simulink model "Testing"  (R2018b)
settings: Solver=VariableStepAuto  StartTime=0.0  StopTime=10.0  RelTol=1e-3
undefined symbols (not defined in the file): BattTempBp, BM_TiCtctrCnct_P, BM_TiCtctrDCnct_P, BMS_EnaFltSts, BMS_ModeEnaFltChk, BMS_TiSample_C, BPC_BattTotalCharge_P, BPC_BattTotalEnergy_P, CapLUTBp, CapSOCBp, CVM_DMaxVCellMaxCutoff_P, CVM_DMaxVCellMaxDrtd_P, CVM_DMaxVCellMaxWarn_P, CVM_DMaxVCellMinCutoff_P, CVM_DMaxVCellMinDrtd_P, CVM_DMaxVCellMinWarn_P, CVM_DMinVCellMaxCutoff_P, CVM_DMinVCellMaxDrtd_P, CVM_DMinVCellMaxWarn_P, CVM_DMinVCellMinCutoff_P, CVM_DMinVCellMinDrtd_P, CVM_DMinVCellMinWarn_P, CVM_VCellMaxCutoffTh_P, CVM_VCellMaxDrtdTh_P, CVM_VCellMaxWarnTh_P, CVM_VCellMinCutoffTh_P, CVM_VCellMinDrtdTh_P, CVM_VCellMinWarnTh_P, DiscIntNeverNeededParam, Em, MTM_DMaxTMdulMaxCutoff_P, MTM_DMaxTMdulMaxDrtd_P, MTM_DMaxTMdulMaxWarn_P, MTM_DMaxTMdulMinCutoff_P, MTM_DMaxTMdulMinDrtd_P, MTM_DMaxTMdulMinWarn_P, MTM_DMinTMdulMaxCutoff_P, MTM_DMinTMdulMaxDrtd_P, MTM_DMinTMdulMaxWarn_P, MTM_DMinTMdulMinCutoff_P, MTM_DMinTMdulMinDrtd_P, MTM_DMinTMdulMinWarn_P, MTM_TMdulMaxCutoffTh_P, MTM_TMdulMaxDrtdTh_P, MTM_TMdulMaxWarnTh_P, MTM_TMdulMinCutoffTh_P, MTM_TMdulMinDrtdTh_P, MTM_TMdulMinWarnTh_P, NrCutoff_C, NrDrtd_C, NrNoFlt_C, NrTMdulSnsr_C, NrWarn_C, RInt
libraries: BMSLib x12
settings Model: Creator=Administrator  LastModifiedBy=Administrator
settings OptimizationCC: DefaultUnderspecifiedDataType=single

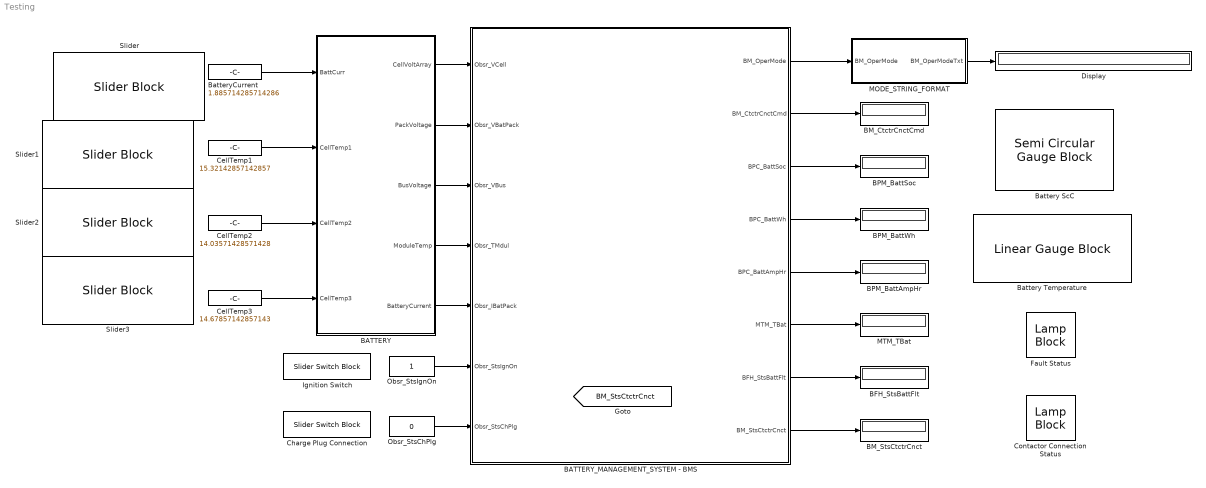
== system Testing ==
  BATTERY : Subsystem
  BATTERY_MANAGEMENT_SYSTEM - BMS : Subsystem
  BFH_StsBattFlt : Display
  BM_CtctrCnctCmd : Display
  BM_StsCtctrCnct : Display
  BPM_BattAmpHr : Display
  BPM_BattSoc : Display
  BPM_BattWh : Display
  Battery ScC : SemiCircularGaugeBlock  WebBlockId=770
  Battery Temperature : LinearGaugeBlock  WebBlockId=771  ScaleMin=-60  ScaleMax=60
  BatteryCurrent : Constant  Value=1.885714285714286  OutDataTypeStr=double
  CellTemp1 : Constant  Value=15.32142857142857  OutDataTypeStr=double
  CellTemp2 : Constant  Value=14.03571428571428  OutDataTypeStr=double
  CellTemp3 : Constant  Value=14.67857142857143  OutDataTypeStr=double
  Charge Plug Connection : SliderSwitchBlock  WebBlockId=776
      settings: Values={{'Off', 'On'}, [0 1]}
  Contactor Connection Status : LampBlock  WebBlockId=777
  Display : Display
  Fault Status : LampBlock  WebBlockId=779
  Ignition Switch : SliderSwitchBlock  WebBlockId=781
      settings: Values={{'Off', 'On'}, [0 1]}
  MODE_STRING_FORMAT : Subsystem
  MTM_TBat : Display
  Obsr_StsChPlg : Constant  Value=0  OutDataTypeStr=boolean
  Obsr_StsIgnOn : Constant  OutDataTypeStr=boolean
  Slider : SliderBlock  WebBlockId=791  ScaleMin=-24  ScaleMax=24
  Slider1 : SliderBlock  WebBlockId=792  ScaleMin=-30  ScaleMax=60
  Slider2 : SliderBlock  WebBlockId=793  ScaleMin=-30  ScaleMax=60
  Slider3 : SliderBlock  WebBlockId=794  ScaleMin=-30  ScaleMax=60
  tag scope: BM_StsCtctrCnct=global
  wires:
  Obsr_StsChPlg/1 -> BATTERY_MANAGEMENT_SYSTEM - BMS/7(Obsr_StsChPlg)
  BATTERY_MANAGEMENT_SYSTEM - BMS/2(BM_CtctrCnctCmd) -> BM_CtctrCnctCmd/1
  BATTERY_MANAGEMENT_SYSTEM - BMS/3(BPC_BattSoc) -> BPM_BattSoc/1
  BatteryCurrent/1 -> BATTERY/1(BattCurr)
  Obsr_StsIgnOn/1 -> BATTERY_MANAGEMENT_SYSTEM - BMS/6(Obsr_StsIgnOn)
  MODE_STRING_FORMAT/1(BM_OperModeTxt) -> Display/1
  BATTERY/2(PackVoltage) -> BATTERY_MANAGEMENT_SYSTEM - BMS/2(Obsr_VBatPack)
  BATTERY_MANAGEMENT_SYSTEM - BMS/1(BM_OperMode) -> MODE_STRING_FORMAT/1(BM_OperMode)
  BATTERY_MANAGEMENT_SYSTEM - BMS/4(BPC_BattWh) -> BPM_BattWh/1
  BATTERY_MANAGEMENT_SYSTEM - BMS/5(BPC_BattAmpHr) -> BPM_BattAmpHr/1
  CellTemp1/1 -> BATTERY/2(CellTemp1)
  BATTERY/5(BatteryCurrent) -> BATTERY_MANAGEMENT_SYSTEM - BMS/5(Obsr_IBatPack)
  BATTERY/4(ModuleTemp) -> BATTERY_MANAGEMENT_SYSTEM - BMS/4(Obsr_TMdul)
  CellTemp3/1 -> BATTERY/4(CellTemp3)
  CellTemp2/1 -> BATTERY/3(CellTemp2)
  BATTERY/1(CellVoltArray) -> BATTERY_MANAGEMENT_SYSTEM - BMS/1(Obsr_VCell)
  BATTERY_MANAGEMENT_SYSTEM - BMS/6(MTM_TBat) -> MTM_TBat/1
  BATTERY_MANAGEMENT_SYSTEM - BMS/7(BFH_StsBattFlt) -> BFH_StsBattFlt/1
  BATTERY/3(BusVoltage) -> BATTERY_MANAGEMENT_SYSTEM - BMS/3(Obsr_VBus)
  BATTERY_MANAGEMENT_SYSTEM - BMS/8(BM_StsCtctrCnct) -> BM_StsCtctrCnct/1

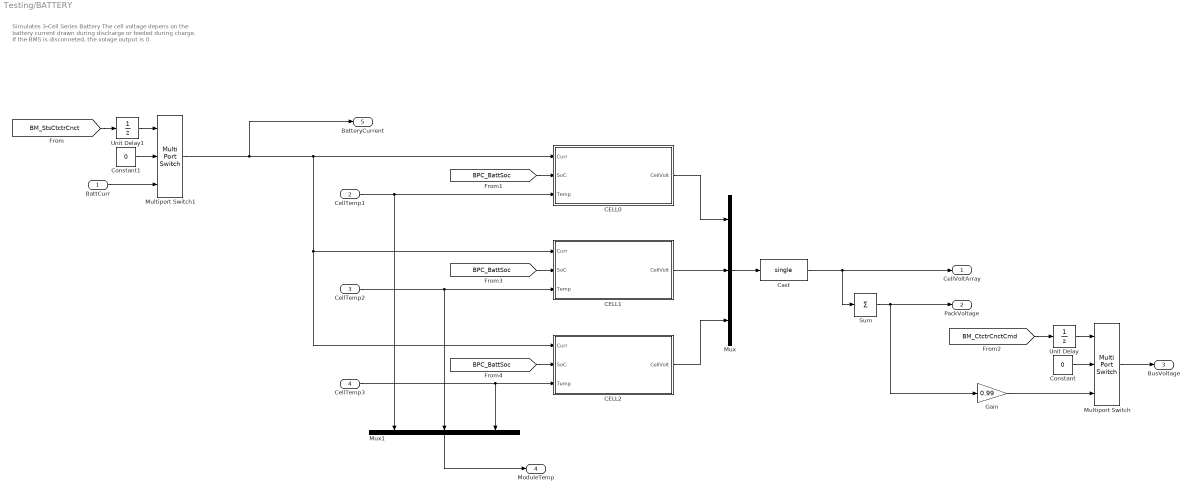
== system Testing/BATTERY ==
  note: Simulates 3-Cell Series Battery
      |
      | The cell voltage depens on the battery current drawn during discharge or feeded during charge.
      |
      | If the BMS is disconneted, the volage output is 0.
  BattCurr : Inport
  CellTemp1 : Inport  Port=2
  CellTemp2 : Inport  Port=3
  CellTemp3 : Inport  Port=4
  CELL0 : Subsystem
  CELL1 : Subsystem
  CELL2 : Subsystem
  Cast : DataTypeConversion  OutDataTypeStr=single
  Constant : Constant  Value=0
  Constant1 : Constant  Value=0
  Gain : Gain  Gain=0.99  OutDataTypeStr=single
  Multiport Switch : MultiPortSwitch  DataPortOrder=Zero-based contiguous  Inputs=2  zeroidx=on  OutDataTypeStr=single
  Multiport Switch1 : MultiPortSwitch  DataPortOrder=Zero-based contiguous  Inputs=2  zeroidx=on
  Mux : Mux  Inputs=3
  Mux1 : Mux  Inputs=3
  Sum : Sum  Inputs=1  AccumDataTypeStr=single
  Unit Delay : UnitDelay  SampleTime=-1
  Unit Delay1 : UnitDelay  SampleTime=-1
  CellVoltArray : Outport
  PackVoltage : Outport  Port=2
  BusVoltage : Outport  Port=3
  ModuleTemp : Outport  Port=4
  BatteryCurrent : Outport  Port=5
  wires:
  CellTemp2/1 -> CELL1/3(Temp), Mux1/2
  CELL1/1(CellVolt) -> Mux/2
  CellTemp3/1 -> CELL2/3(Temp), Mux1/3
  CELL0/1(CellVolt) -> Mux/1
  CellTemp1/1 -> CELL0/3(Temp), Mux1/1
  Mux/1 -> Cast/1
  Sum/1 -> PackVoltage/1, Gain/1
  Mux1/1 -> ModuleTemp/1
  Cast/1 -> Sum/1, CellVoltArray/1
  Multiport Switch1/1 -> CELL0/1(Curr), CELL2/1(Curr), CELL1/1(Curr), BatteryCurrent/1
  Unit Delay/1 -> Multiport Switch/1
  [BM_CtctrCnctCmd] -> Unit Delay/1
  Multiport Switch/1 -> BusVoltage/1
  Gain/1 -> Multiport Switch/3
  Constant/1 -> Multiport Switch/2
  Unit Delay1/1 -> Multiport Switch1/1
  [BM_StsCtctrCnct] -> Unit Delay1/1
  Constant1/1 -> Multiport Switch1/2
  BattCurr/1 -> Multiport Switch1/3
  [BPC_BattSoc] -> CELL0/2(SoC)
  [BPC_BattSoc] -> CELL1/2(SoC)
  [BPC_BattSoc] -> CELL2/2(SoC)
  CELL2/1(CellVolt) -> Mux/3

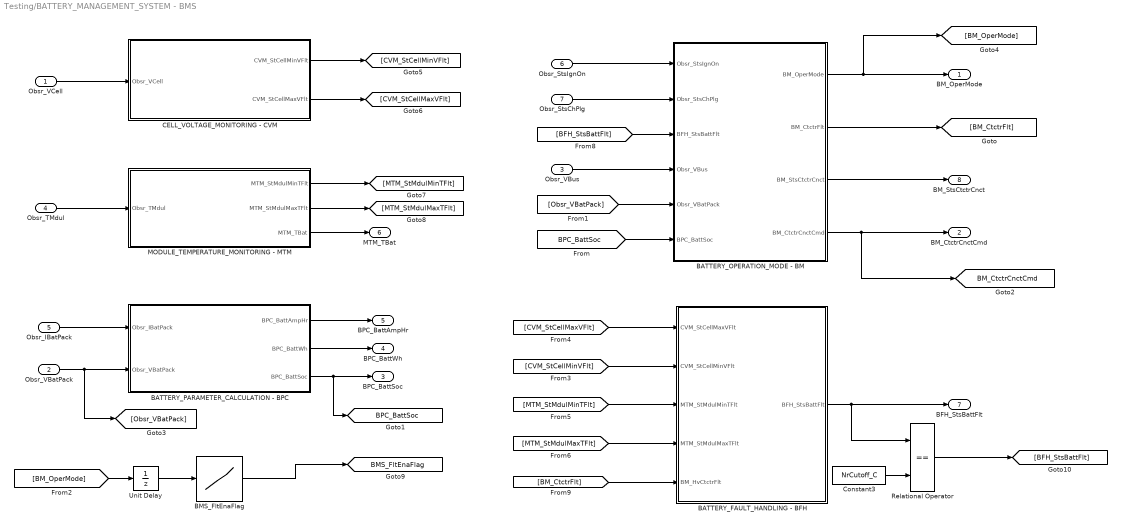
== system Testing/BATTERY_MANAGEMENT_SYSTEM - BMS ==
  Obsr_VCell : Inport
  Obsr_VBatPack : Inport  Port=2
  Obsr_VBus : Inport  Port=3
  Obsr_TMdul : Inport  Port=4
  Obsr_IBatPack : Inport  Port=5
  Obsr_StsIgnOn : Inport  Port=6
  Obsr_StsChPlg : Inport  Port=7
  BATTERY_FAULT_HANDLING - BFH : Subsystem
  BATTERY_OPERATION_MODE - BM : Subsystem
  BATTERY_PARAMETER_CALCULATION - BPC : Subsystem
  BMS_FltEnaFlag : Lookup_n-D  NumberOfTableDimensions=1  BreakpointsForDimension1=BMS_ModeEnaFltChk  Table=BMS_EnaFltSts  InterpMethod=Nearest  ExtrapMethod=Clip  DiagnosticForOutOfRangeInput=Error  InternalRulePriority=Speed  RndMeth=Simplest  InputSameDT=on
  CELL_VOLTAGE_MONITORING - CVM : Subsystem
  Constant3 : Constant  Value=NrCutoff_C
  MODULE_TEMPERATURE_MONITORING - MTM : Subsystem
  Relational Operator : RelationalOperator  Operator===  OutDataTypeStr=boolean  RndMeth=Simplest
  Unit Delay : UnitDelay  SampleTime=-1
  BM_OperMode : Outport
  BM_CtctrCnctCmd : Outport  Port=2
  BPC_BattSoc : Outport  Port=3
  BPC_BattWh : Outport  Port=4
  BPC_BattAmpHr : Outport  Port=5
  MTM_TBat : Outport  Port=6
  BFH_StsBattFlt : Outport  Port=7
  BM_StsCtctrCnct : Outport  Port=8
  tag scope: BMS_FltEnaFlag=global, BM_CtctrCnctCmd=global, BPC_BattSoc=global
  wires:
  Obsr_VCell/1 -> CELL_VOLTAGE_MONITORING - CVM/1(Obsr_VCell)
  Obsr_TMdul/1 -> MODULE_TEMPERATURE_MONITORING - MTM/1(Obsr_TMdul)
  [BPC_BattSoc] -> BATTERY_OPERATION_MODE - BM/6(BPC_BattSoc)
  Obsr_StsIgnOn/1 -> BATTERY_OPERATION_MODE - BM/1(Obsr_StsIgnOn)
  Obsr_StsChPlg/1 -> BATTERY_OPERATION_MODE - BM/2(Obsr_StsChPlg)
  [BFH_StsBattFlt] -> BATTERY_OPERATION_MODE - BM/3(BFH_StsBattFlt)
  Obsr_VBus/1 -> BATTERY_OPERATION_MODE - BM/4(Obsr_VBus)
  BATTERY_OPERATION_MODE - BM/4(BM_CtctrCnctCmd) -> BM_CtctrCnctCmd/1, [BM_CtctrCnctCmd]
  BATTERY_OPERATION_MODE - BM/2(BM_CtctrFlt) -> [BM_CtctrFlt]
  Obsr_VBatPack/1 -> BATTERY_PARAMETER_CALCULATION - BPC/2(Obsr_VBatPack), [Obsr_VBatPack]
  [Obsr_VBatPack] -> BATTERY_OPERATION_MODE - BM/5(Obsr_VBatPack)
  CELL_VOLTAGE_MONITORING - CVM/1(CVM_StCellMinVFlt) -> [CVM_StCellMinVFlt]
  CELL_VOLTAGE_MONITORING - CVM/2(CVM_StCellMaxVFlt) -> [CVM_StCellMaxVFlt]
  MODULE_TEMPERATURE_MONITORING - MTM/1(MTM_StMdulMinTFlt) -> [MTM_StMdulMinTFlt]
  MODULE_TEMPERATURE_MONITORING - MTM/2(MTM_StMdulMaxTFlt) -> [MTM_StMdulMaxTFlt]
  MODULE_TEMPERATURE_MONITORING - MTM/3(MTM_TBat) -> MTM_TBat/1
  [CVM_StCellMaxVFlt] -> BATTERY_FAULT_HANDLING - BFH/1(CVM_StCellMaxVFlt)
  [CVM_StCellMinVFlt] -> BATTERY_FAULT_HANDLING - BFH/2(CVM_StCellMinVFlt)
  [MTM_StMdulMinTFlt] -> BATTERY_FAULT_HANDLING - BFH/3(MTM_StMdulMinTFlt)
  [MTM_StMdulMaxTFlt] -> BATTERY_FAULT_HANDLING - BFH/4(MTM_StMdulMaxTFlt)
  BATTERY_FAULT_HANDLING - BFH/1(BFH_StsBattFlt) -> Relational Operator/1, BFH_StsBattFlt/1
  [BM_CtctrFlt] -> BATTERY_FAULT_HANDLING - BFH/5(BM_HvCtctrFlt)
  BATTERY_OPERATION_MODE - BM/3(BM_StsCtctrCnct) -> BM_StsCtctrCnct/1
  Relational Operator/1 -> [BFH_StsBattFlt]
  Constant3/1 -> Relational Operator/2
  BATTERY_OPERATION_MODE - BM/1(BM_OperMode) -> [BM_OperMode], BM_OperMode/1
  [BM_OperMode] -> Unit Delay/1
  BMS_FltEnaFlag/1 -> [BMS_FltEnaFlag]
  Unit Delay/1 -> BMS_FltEnaFlag/1
  BATTERY_PARAMETER_CALCULATION - BPC/1(BPC_BattAmpHr) -> BPC_BattAmpHr/1
  BATTERY_PARAMETER_CALCULATION - BPC/2(BPC_BattWh) -> BPC_BattWh/1
  BATTERY_PARAMETER_CALCULATION - BPC/3(BPC_BattSoc) -> [BPC_BattSoc], BPC_BattSoc/1
  Obsr_IBatPack/1 -> BATTERY_PARAMETER_CALCULATION - BPC/1(Obsr_IBatPack)

== system Testing/MODE_STRING_FORMAT ==
  BM_OperMode : Inport
  ASCII to String : ASCIIToString
  Cast : DataTypeConversion  OutDataTypeStr=uint8
  MATLAB Function : MATLAB Function  TreatAsAtomicUnit=on
  BM_OperModeTxt : Outport
  wires:
  Cast/1 -> ASCII to String/1
  ASCII to String/1 -> BM_OperModeTxt/1
  MATLAB Function/1(BmsModeText) -> Cast/1
  BM_OperMode/1 -> MATLAB Function/1(ModeNum)

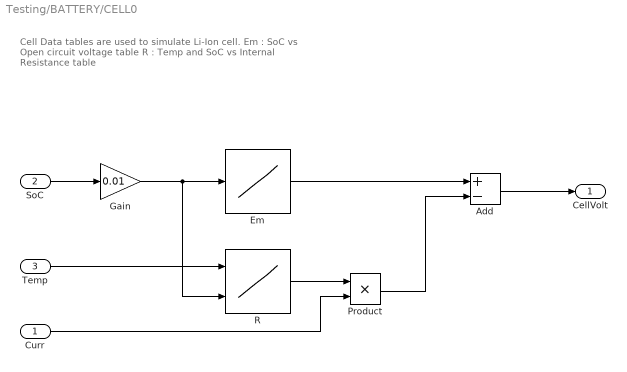
== system Testing/BATTERY/CELL0 ==
  note: Cell
      |
      | Data tables are used to simulate Li-Ion cell.
      |
      | Em : SoC vs Open circuit voltage table
      |
      | R : Temp and SoC vs Internal Resistance table
  Curr : Inport
  SoC : Inport  Port=2
  Temp : Inport  Port=3
  Add : Sum  Inputs=+-
  Em : Lookup_n-D  NumberOfTableDimensions=1  BreakpointsForDimension1=CapLUTBp  Table=Em  ExtrapMethod=Clip  UseLastTableValue=on  InternalRulePriority=Speed  RndMeth=Simplest  InputSameDT=on
  Gain : Gain  Gain=0.01  OutDataTypeStr=double
  Product : Product
  R : Lookup_n-D  BreakpointsForDimension1=BattTempBp  BreakpointsForDimension2=CapSOCBp  Table=RInt  ExtrapMethod=Clip  UseLastTableValue=on  InternalRulePriority=Speed  RndMeth=Simplest  InputSameDT=on
  CellVolt : Outport
  wires:
  SoC/1 -> Gain/1
  Product/1 -> Add/2
  Curr/1 -> Product/2
  Add/1 -> CellVolt/1
  Temp/1 -> R/1
  R/1 -> Product/1
  Em/1 -> Add/1
  Gain/1 -> R/2, Em/1

== system Testing/BATTERY/CELL1 ==
  note: Cell
      |
      | Data tables are used to simulate Li-Ion cell.
      |
      | Em : SoC vs Open circuit voltage table
      |
      | R : Temp and SoC vs Internal Resistance table
  Curr : Inport
  SoC : Inport  Port=2
  Temp : Inport  Port=3
  Add : Sum  Inputs=+-
  Em : Lookup_n-D  NumberOfTableDimensions=1  BreakpointsForDimension1=CapLUTBp  Table=Em  InternalRulePriority=Speed  RndMeth=Simplest  InputSameDT=on
  Gain : Gain  Gain=0.01  OutDataTypeStr=double
  Product : Product
  R : Lookup_n-D  BreakpointsForDimension1=BattTempBp  BreakpointsForDimension2=CapSOCBp  Table=RInt  InternalRulePriority=Speed  RndMeth=Simplest  InputSameDT=on
  CellVolt : Outport
  wires:
  Gain/1 -> Em/1, R/2
  Em/1 -> Add/1
  R/1 -> Product/1
  Temp/1 -> R/1
  Add/1 -> CellVolt/1
  Curr/1 -> Product/2
  Product/1 -> Add/2
  SoC/1 -> Gain/1

== system Testing/BATTERY/CELL2 ==
  note: Cell
      |
      | Data tables are used to simulate Li-Ion cell.
      |
      | Em : SoC vs Open circuit voltage table
      |
      | R : Temp and SoC vs Internal Resistance table
  Curr : Inport
  SoC : Inport  Port=2
  Temp : Inport  Port=3
  Add : Sum  Inputs=+-
  Em : Lookup_n-D  NumberOfTableDimensions=1  BreakpointsForDimension1=CapLUTBp  Table=Em  InternalRulePriority=Speed  RndMeth=Simplest  InputSameDT=on
  Gain : Gain  Gain=0.01  OutDataTypeStr=double
  Product : Product
  R : Lookup_n-D  BreakpointsForDimension1=BattTempBp  BreakpointsForDimension2=CapSOCBp  Table=RInt  InternalRulePriority=Speed  RndMeth=Simplest  InputSameDT=on
  CellVolt : Outport
  wires:
  SoC/1 -> Gain/1
  Product/1 -> Add/2
  Curr/1 -> Product/2
  Add/1 -> CellVolt/1
  Temp/1 -> R/1
  R/1 -> Product/1
  Em/1 -> Add/1
  Gain/1 -> R/2, Em/1

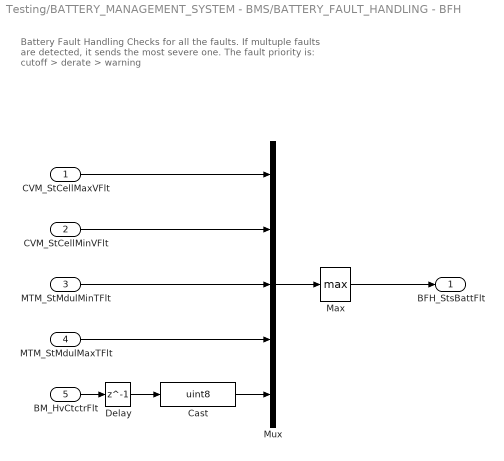
== system Testing/BATTERY_MANAGEMENT_SYSTEM - BMS/BATTERY_FAULT_HANDLING - BFH ==
  note: Battery Fault Handling
      |
      | Checks for all the faults. If multuple faults are detected, it sends the most severe one.
      |
      | The fault priority is: cutoff > derate > warning
  CVM_StCellMaxVFlt : Inport
  CVM_StCellMinVFlt : Inport  Port=2
  MTM_StMdulMinTFlt : Inport  Port=3
  MTM_StMdulMaxTFlt : Inport  Port=4
  BM_HvCtctrFlt : Inport  Port=5
  Cast : DataTypeConversion  OutDataTypeStr=uint8
  Delay : Delay  DelayLength=1
  Max : MinMax  Function=max  OutDataTypeStr=uint8
  Mux : Mux  Inputs=5
  BFH_StsBattFlt : Outport
  wires:
  Mux/1 -> Max/1
  MTM_StMdulMaxTFlt/1 -> Mux/4
  CVM_StCellMinVFlt/1 -> Mux/2
  CVM_StCellMaxVFlt/1 -> Mux/1
  MTM_StMdulMinTFlt/1 -> Mux/3
  Max/1 -> BFH_StsBattFlt/1
  BM_HvCtctrFlt/1 -> Delay/1
  Cast/1 -> Mux/5
  Delay/1 -> Cast/1

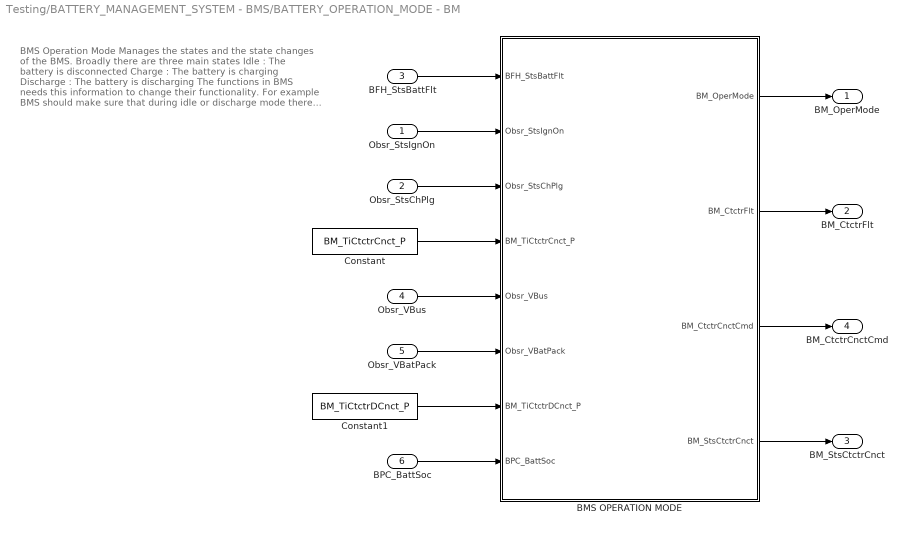
== system Testing/BATTERY_MANAGEMENT_SYSTEM - BMS/BATTERY_OPERATION_MODE - BM ==
  note: BMS Operation Mode
      |
      | Manages the states and the state changes of the BMS. Broadly there are three main states
      | Idle : The battery is disconnected
      | Charge : The battery is charging
      | Discharge : The battery is discharging
      |
      | The functions in BMS needs this information to change their functionality. For example BMS should make sure that during idle or discharge mode there is no current going into the battery. The SoC should increase during charge and decrease during discharge.
  Obsr_StsIgnOn : Inport
  Obsr_StsChPlg : Inport  Port=2
  BFH_StsBattFlt : Inport  Port=3
  Obsr_VBus : Inport  Port=4
  Obsr_VBatPack : Inport  Port=5
  BPC_BattSoc : Inport  Port=6
  BMS OPERATION MODE : Stateflow chart  TreatAsAtomicUnit=on
  Constant : Constant  Value=BM_TiCtctrCnct_P
  Constant1 : Constant  Value=BM_TiCtctrDCnct_P
  BM_OperMode : Outport
  BM_CtctrFlt : Outport  Port=2
  BM_StsCtctrCnct : Outport  Port=3
  BM_CtctrCnctCmd : Outport  Port=4
  wires:
  BFH_StsBattFlt/1 -> BMS OPERATION MODE/1(BFH_StsBattFlt)
  Obsr_StsIgnOn/1 -> BMS OPERATION MODE/2(Obsr_StsIgnOn)
  Obsr_StsChPlg/1 -> BMS OPERATION MODE/3(Obsr_StsChPlg)
  Obsr_VBus/1 -> BMS OPERATION MODE/5(Obsr_VBus)
  Obsr_VBatPack/1 -> BMS OPERATION MODE/6(Obsr_VBatPack)
  Constant/1 -> BMS OPERATION MODE/4(BM_TiCtctrCnct_P)
  Constant1/1 -> BMS OPERATION MODE/7(BM_TiCtctrDCnct_P)
  BMS OPERATION MODE/1(BM_OperMode) -> BM_OperMode/1
  BMS OPERATION MODE/2(BM_CtctrFlt) -> BM_CtctrFlt/1
  BMS OPERATION MODE/4(BM_StsCtctrCnct) -> BM_StsCtctrCnct/1
  BMS OPERATION MODE/3(BM_CtctrCnctCmd) -> BM_CtctrCnctCmd/1
  BPC_BattSoc/1 -> BMS OPERATION MODE/8(BPC_BattSoc)

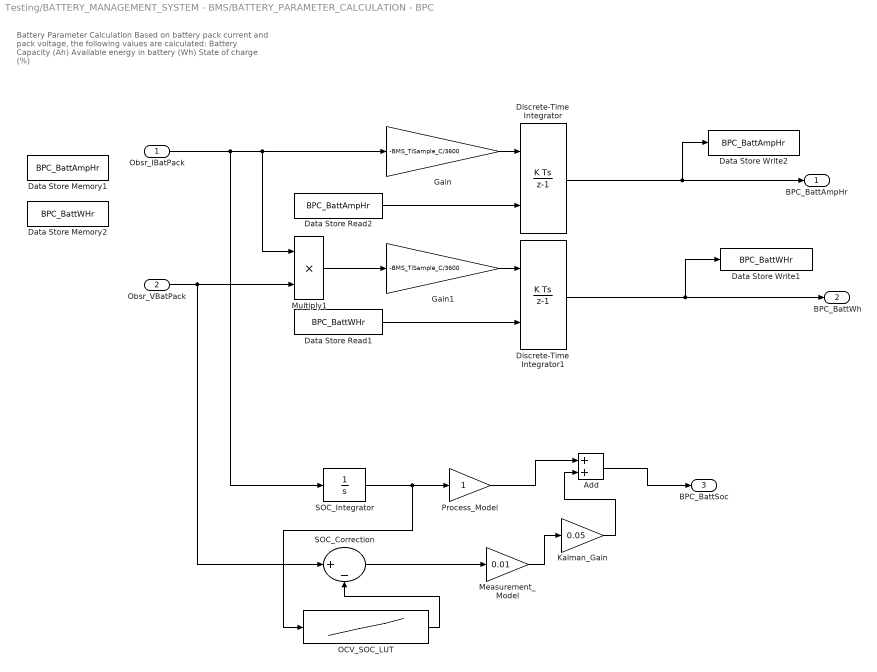
== system Testing/BATTERY_MANAGEMENT_SYSTEM - BMS/BATTERY_PARAMETER_CALCULATION - BPC ==
  note: Battery Parameter Calculation
      |
      | Based on battery pack current and pack voltage, the following values are calculated:
      | Battery Capacity (Ah)
      | Available energy in battery (Wh)
      | State of charge (%)
  Obsr_IBatPack : Inport
  Obsr_VBatPack : Inport  Port=2
  Add : Sum
  Data Store Memory1 : DataStoreMemory  DataStoreName=BPC_BattAmpHr  ReadBeforeWriteMsg=warning  WriteAfterWriteMsg=warning  WriteAfterReadMsg=warning  InitialValue=48*0.985  ShowAdditionalParam=off  OutDataTypeStr=double
  Data Store Memory2 : DataStoreMemory  DataStoreName=BPC_BattWHr  ReadBeforeWriteMsg=warning  WriteAfterWriteMsg=warning  WriteAfterReadMsg=warning  InitialValue=48*3*4.22*0.985  ShowAdditionalParam=off  OutDataTypeStr=double
  Data Store Read1 : DataStoreRead  DataStoreName=BPC_BattWHr
  Data Store Read2 : DataStoreRead  DataStoreName=BPC_BattAmpHr
  Data Store Write1 : DataStoreWrite  DataStoreName=BPC_BattWHr
  Data Store Write2 : DataStoreWrite  DataStoreName=BPC_BattAmpHr
  Discrete-Time Integrator : DiscreteIntegrator  InitialConditionSource=external  SampleTime=-1  LimitOutput=on  UpperSaturationLimit=BPC_BattTotalCharge_P  LowerSaturationLimit=0  ICPrevOutput=DiscIntNeverNeededParam  ICPrevScaledInput=DiscIntNeverNeededParam
  Discrete-Time Integrator1 : DiscreteIntegrator  InitialConditionSource=external  SampleTime=-1  LimitOutput=on  UpperSaturationLimit=BPC_BattTotalEnergy_P  LowerSaturationLimit=0  ICPrevOutput=DiscIntNeverNeededParam  ICPrevScaledInput=DiscIntNeverNeededParam
  Gain : Gain  Gain=-BMS_TiSample_C/3600  OutDataTypeStr=double
  Gain1 : Gain  Gain=-BMS_TiSample_C/3600  OutDataTypeStr=double
  Kalman_Gain : Gain  Gain=0.05
  Measurement_Model : Gain  Gain=0.01
  Multiply1 : Product
  OCV_SOC_LUT : Lookup_n-D  NumberOfTableDimensions=1  BreakpointsForDimension1=[-5:5]  Table=tanh([-5:5])  InternalRulePriority=Speed  RndMeth=Simplest  InputSameDT=on
  Process_Model : Gain
  SOC_Correction : Sum  Inputs=|+-
  SOC_Integrator : Integrator
  BPC_BattAmpHr : Outport
  BPC_BattWh : Outport  Port=2
  BPC_BattSoc : Outport  Port=3
  wires:
  Add/1 -> BPC_BattSoc/1
  Process_Model/1 -> Add/1
  Data Store Read2/1 -> Discrete-Time Integrator/2
  Discrete-Time Integrator1/1 -> Data Store Write1/1, BPC_BattWh/1
  SOC_Correction/1 -> Measurement_Model/1
  Discrete-Time Integrator/1 -> Data Store Write2/1, BPC_BattAmpHr/1
  Data Store Read1/1 -> Discrete-Time Integrator1/2
  Gain/1 -> Discrete-Time Integrator/1
  Obsr_IBatPack/1 -> SOC_Integrator/1, Multiply1/1, Gain/1
  Multiply1/1 -> Gain1/1
  OCV_SOC_LUT/1 -> SOC_Correction/2
  SOC_Integrator/1 -> OCV_SOC_LUT/1, Process_Model/1
  Measurement_Model/1 -> Kalman_Gain/1
  Kalman_Gain/1 -> Add/2
  Gain1/1 -> Discrete-Time Integrator1/1
  Obsr_VBatPack/1 -> SOC_Correction/1, Multiply1/2

== system Testing/BATTERY_MANAGEMENT_SYSTEM - BMS/CELL_VOLTAGE_MONITORING - CVM ==
  note: Cell Voltage Monitoring
      |
      | Checks for cell over-voltage and under-voltage faults
  Obsr_VCell : Inport
  Max_Cell_Voltage_Fault_State : Subsystem
  Min : MinMax
  Min1 : MinMax  Function=max
  Min_Cell_Voltage_Fault_State : Subsystem
  CVM_StCellMinVFlt : Outport
  CVM_StCellMaxVFlt : Outport  Port=2
  wires:
  Obsr_VCell/1 -> Min/1, Min1/1
  Min/1 -> Min_Cell_Voltage_Fault_State/1(CVM_VCellMin)
  Min1/1 -> Max_Cell_Voltage_Fault_State/1(CVM_VCellMin)
  Min_Cell_Voltage_Fault_State/1(CVM_StCellMinVFlt) -> CVM_StCellMinVFlt/1
  Max_Cell_Voltage_Fault_State/1(CVM_StCellMaxVFlt) -> CVM_StCellMaxVFlt/1

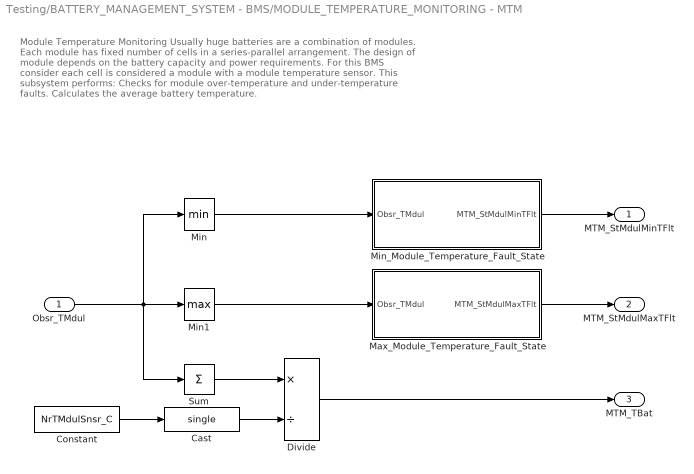
== system Testing/BATTERY_MANAGEMENT_SYSTEM - BMS/MODULE_TEMPERATURE_MONITORING - MTM ==
  note: Module Temperature Monitoring
      |
      | Usually huge batteries are a combination of modules. Each module has fixed number of cells in a series-parallel arrangement. The design of module depends on the battery capacity and power requirements. For this BMS consider each cell is considered a module with a module temperature sensor. This subsystem performs:
      |
      | Checks for module over-temperature and under-temperature faults.
      |
      | Calculates the average battery temperature.
  Obsr_TMdul : Inport
  Cast : DataTypeConversion  OutDataTypeStr=single
  Constant : Constant  Value=NrTMdulSnsr_C
  Divide : Product  Inputs=*/
  Max_Module_Temperature_Fault_State : Subsystem
  Min : MinMax
  Min1 : MinMax  Function=max
  Min_Module_Temperature_Fault_State : Subsystem
  Sum : Sum  Inputs=+
  MTM_StMdulMinTFlt : Outport
  MTM_StMdulMaxTFlt : Outport  Port=2
  MTM_TBat : Outport  Port=3
  wires:
  Min1/1 -> Max_Module_Temperature_Fault_State/1(Obsr_TMdul)
  Max_Module_Temperature_Fault_State/1(MTM_StMdulMaxTFlt) -> MTM_StMdulMaxTFlt/1
  Min/1 -> Min_Module_Temperature_Fault_State/1(Obsr_TMdul)
  Min_Module_Temperature_Fault_State/1(MTM_StMdulMinTFlt) -> MTM_StMdulMinTFlt/1
  Obsr_TMdul/1 -> Min/1, Sum/1, Min1/1
  Sum/1 -> Divide/1
  Divide/1 -> MTM_TBat/1
  Constant/1 -> Cast/1
  Cast/1 -> Divide/2

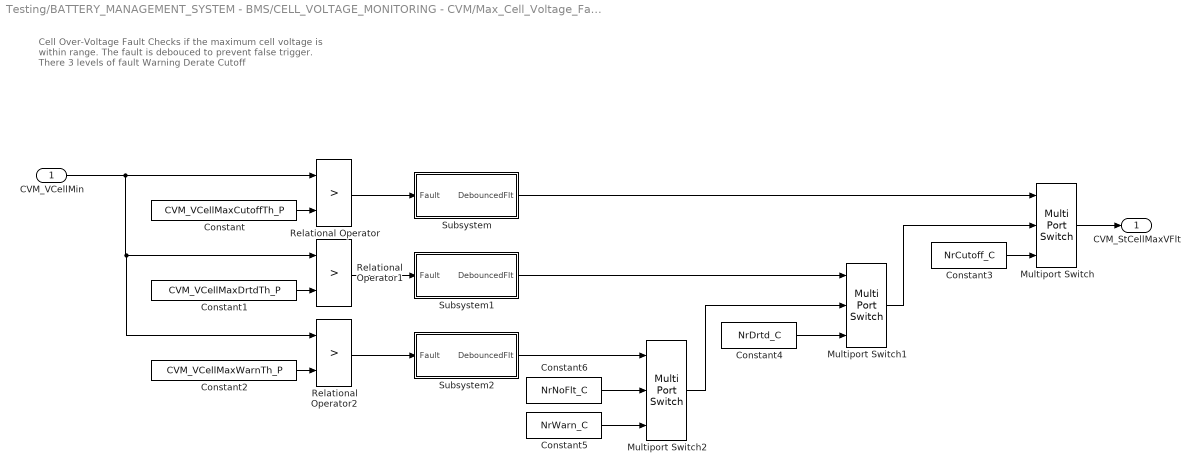
== system Testing/BATTERY_MANAGEMENT_SYSTEM - BMS/CELL_VOLTAGE_MONITORING - CVM/Max_Cell_Voltage_Fault_State ==
  note: Cell Over-Voltage Fault
      |
      | Checks if the maximum cell voltage is within range. The fault is debouced to prevent false trigger.
      |
      | There 3 levels of fault
      | Warning
      | Derate
      | Cutoff
  CVM_VCellMin : Inport
  Constant : Constant  Value=CVM_VCellMaxCutoffTh_P
  Constant1 : Constant  Value=CVM_VCellMaxDrtdTh_P
  Constant2 : Constant  Value=CVM_VCellMaxWarnTh_P
  Constant3 : Constant  Value=NrCutoff_C
  Constant4 : Constant  Value=NrDrtd_C
  Constant5 : Constant  Value=NrWarn_C
  Constant6 : Constant  Value=NrNoFlt_C
  Multiport Switch : MultiPortSwitch  DataPortOrder=Zero-based contiguous  Inputs=2  zeroidx=on
  Multiport Switch1 : MultiPortSwitch  DataPortOrder=Zero-based contiguous  Inputs=2  zeroidx=on
  Multiport Switch2 : MultiPortSwitch  DataPortOrder=Zero-based contiguous  Inputs=2  zeroidx=on
  Relational Operator : RelationalOperator  Operator=>  OutDataTypeStr=boolean  RndMeth=Simplest
  Relational Operator1 : RelationalOperator  Operator=>  OutDataTypeStr=boolean  RndMeth=Simplest
  Relational Operator2 : RelationalOperator  Operator=>  OutDataTypeStr=boolean  RndMeth=Simplest
  Subsystem : Subsystem
  Subsystem1 : Subsystem
  Subsystem2 : Subsystem
  CVM_StCellMaxVFlt : Outport
  wires:
  Constant6/1 -> Multiport Switch2/2
  Constant5/1 -> Multiport Switch2/3
  Constant2/1 -> Relational Operator2/2
  Multiport Switch2/1 -> Multiport Switch1/2
  Constant4/1 -> Multiport Switch1/3
  Constant1/1 -> Relational Operator1/2
  Constant3/1 -> Multiport Switch/3
  Multiport Switch1/1 -> Multiport Switch/2
  Constant/1 -> Relational Operator/2
  Multiport Switch/1 -> CVM_StCellMaxVFlt/1
  CVM_VCellMin/1 -> Relational Operator/1, Relational Operator1/1, Relational Operator2/1
  Relational Operator2/1 -> Subsystem2/1(Fault)
  Subsystem/1(DebouncedFlt) -> Multiport Switch/1
  Relational Operator/1 -> Subsystem/1(Fault)
  Relational Operator1/1 -> Subsystem1/1(Fault)
  Subsystem1/1(DebouncedFlt) -> Multiport Switch1/1
  Subsystem2/1(DebouncedFlt) -> Multiport Switch2/1

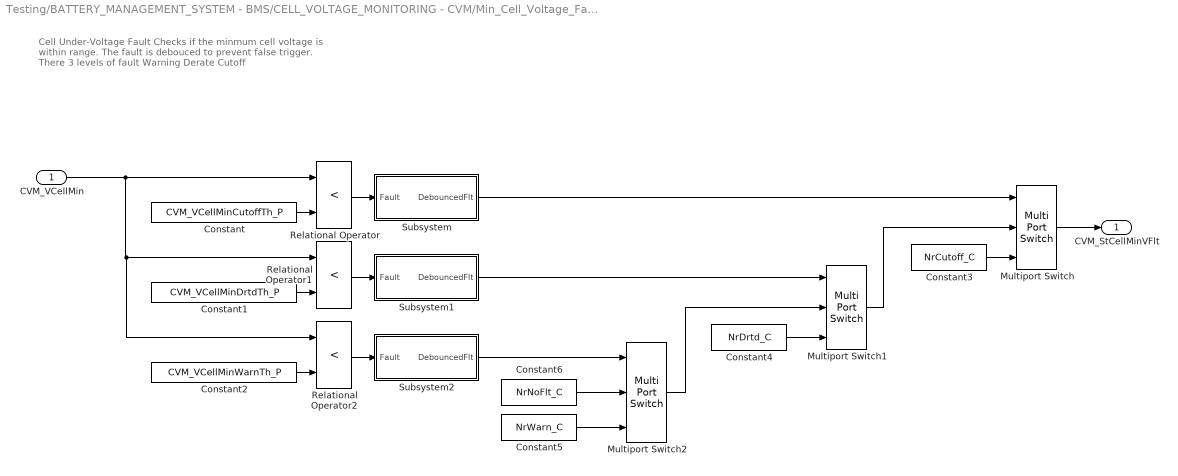
== system Testing/BATTERY_MANAGEMENT_SYSTEM - BMS/CELL_VOLTAGE_MONITORING - CVM/Min_Cell_Voltage_Fault_State ==
  note: Cell Under-Voltage Fault
      |
      | Checks if the minmum cell voltage is within range. The fault is debouced to prevent false trigger.
      |
      | There 3 levels of fault
      | Warning
      | Derate
      | Cutoff
  CVM_VCellMin : Inport
  Constant : Constant  Value=CVM_VCellMinCutoffTh_P
  Constant1 : Constant  Value=CVM_VCellMinDrtdTh_P
  Constant2 : Constant  Value=CVM_VCellMinWarnTh_P
  Constant3 : Constant  Value=NrCutoff_C
  Constant4 : Constant  Value=NrDrtd_C
  Constant5 : Constant  Value=NrWarn_C
  Constant6 : Constant  Value=NrNoFlt_C
  Multiport Switch : MultiPortSwitch  DataPortOrder=Zero-based contiguous  Inputs=2  zeroidx=on
  Multiport Switch1 : MultiPortSwitch  DataPortOrder=Zero-based contiguous  Inputs=2  zeroidx=on
  Multiport Switch2 : MultiPortSwitch  DataPortOrder=Zero-based contiguous  Inputs=2  zeroidx=on
  Relational Operator : RelationalOperator  Operator=<  OutDataTypeStr=boolean  RndMeth=Simplest
  Relational Operator1 : RelationalOperator  Operator=<  OutDataTypeStr=boolean  RndMeth=Simplest
  Relational Operator2 : RelationalOperator  Operator=<  OutDataTypeStr=boolean  RndMeth=Simplest
  Subsystem : Subsystem
  Subsystem1 : Subsystem
  Subsystem2 : Subsystem
  CVM_StCellMinVFlt : Outport
  wires:
  CVM_VCellMin/1 -> Relational Operator2/1, Relational Operator1/1, Relational Operator/1
  Multiport Switch/1 -> CVM_StCellMinVFlt/1
  Relational Operator/1 -> Subsystem/1(Fault)
  Constant/1 -> Relational Operator/2
  Multiport Switch1/1 -> Multiport Switch/2
  Constant3/1 -> Multiport Switch/3
  Relational Operator1/1 -> Subsystem1/1(Fault)
  Constant1/1 -> Relational Operator1/2
  Constant4/1 -> Multiport Switch1/3
  Multiport Switch2/1 -> Multiport Switch1/2
  Relational Operator2/1 -> Subsystem2/1(Fault)
  Constant2/1 -> Relational Operator2/2
  Constant5/1 -> Multiport Switch2/3
  Constant6/1 -> Multiport Switch2/2
  Subsystem/1(DebouncedFlt) -> Multiport Switch/1
  Subsystem1/1(DebouncedFlt) -> Multiport Switch1/1
  Subsystem2/1(DebouncedFlt) -> Multiport Switch2/1

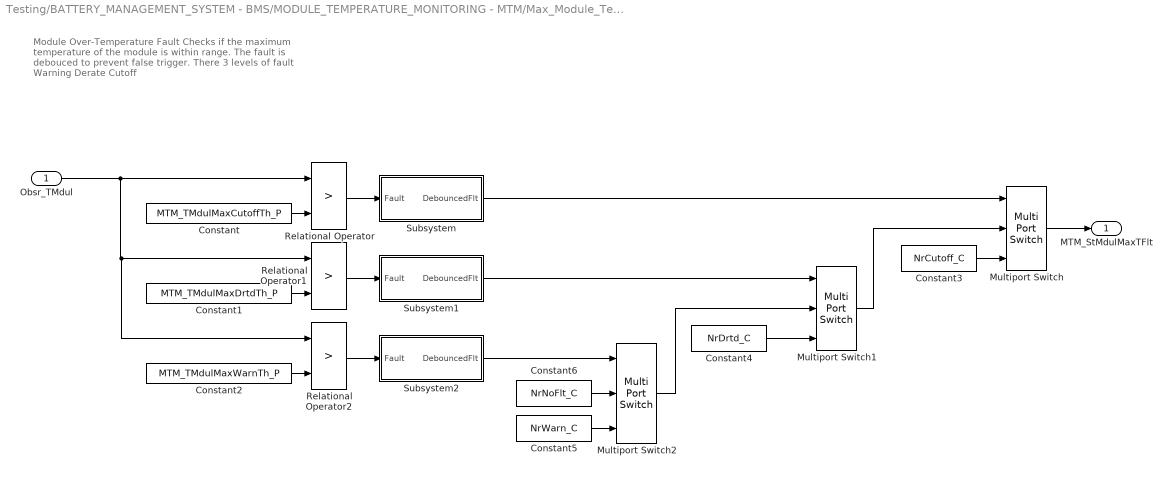
== system Testing/BATTERY_MANAGEMENT_SYSTEM - BMS/MODULE_TEMPERATURE_MONITORING - MTM/Max_Module_Temperature_Fault_State ==
  note: Module Over-Temperature Fault
      |
      | Checks if the maximum temperature of the module is within range. The fault is debouced to prevent false trigger.
      |
      | There 3 levels of fault
      | Warning
      | Derate
      | Cutoff
  Obsr_TMdul : Inport
  Constant : Constant  Value=MTM_TMdulMaxCutoffTh_P
  Constant1 : Constant  Value=MTM_TMdulMaxDrtdTh_P
  Constant2 : Constant  Value=MTM_TMdulMaxWarnTh_P
  Constant3 : Constant  Value=NrCutoff_C
  Constant4 : Constant  Value=NrDrtd_C
  Constant5 : Constant  Value=NrWarn_C
  Constant6 : Constant  Value=NrNoFlt_C
  Multiport Switch : MultiPortSwitch  DataPortOrder=Zero-based contiguous  Inputs=2  zeroidx=on
  Multiport Switch1 : MultiPortSwitch  DataPortOrder=Zero-based contiguous  Inputs=2  zeroidx=on
  Multiport Switch2 : MultiPortSwitch  DataPortOrder=Zero-based contiguous  Inputs=2  zeroidx=on
  Relational Operator : RelationalOperator  Operator=>  OutDataTypeStr=boolean  RndMeth=Simplest
  Relational Operator1 : RelationalOperator  Operator=>  OutDataTypeStr=boolean  RndMeth=Simplest
  Relational Operator2 : RelationalOperator  Operator=>  OutDataTypeStr=boolean  RndMeth=Simplest
  Subsystem : Subsystem
  Subsystem1 : Subsystem
  Subsystem2 : Subsystem
  MTM_StMdulMaxTFlt : Outport
  wires:
  Constant6/1 -> Multiport Switch2/2
  Constant5/1 -> Multiport Switch2/3
  Constant2/1 -> Relational Operator2/2
  Relational Operator2/1 -> Subsystem2/1(Fault)
  Multiport Switch2/1 -> Multiport Switch1/2
  Constant4/1 -> Multiport Switch1/3
  Constant1/1 -> Relational Operator1/2
  Relational Operator1/1 -> Subsystem1/1(Fault)
  Constant3/1 -> Multiport Switch/3
  Multiport Switch1/1 -> Multiport Switch/2
  Constant/1 -> Relational Operator/2
  Relational Operator/1 -> Subsystem/1(Fault)
  Multiport Switch/1 -> MTM_StMdulMaxTFlt/1
  Obsr_TMdul/1 -> Relational Operator/1, Relational Operator1/1, Relational Operator2/1
  Subsystem/1(DebouncedFlt) -> Multiport Switch/1
  Subsystem1/1(DebouncedFlt) -> Multiport Switch1/1
  Subsystem2/1(DebouncedFlt) -> Multiport Switch2/1

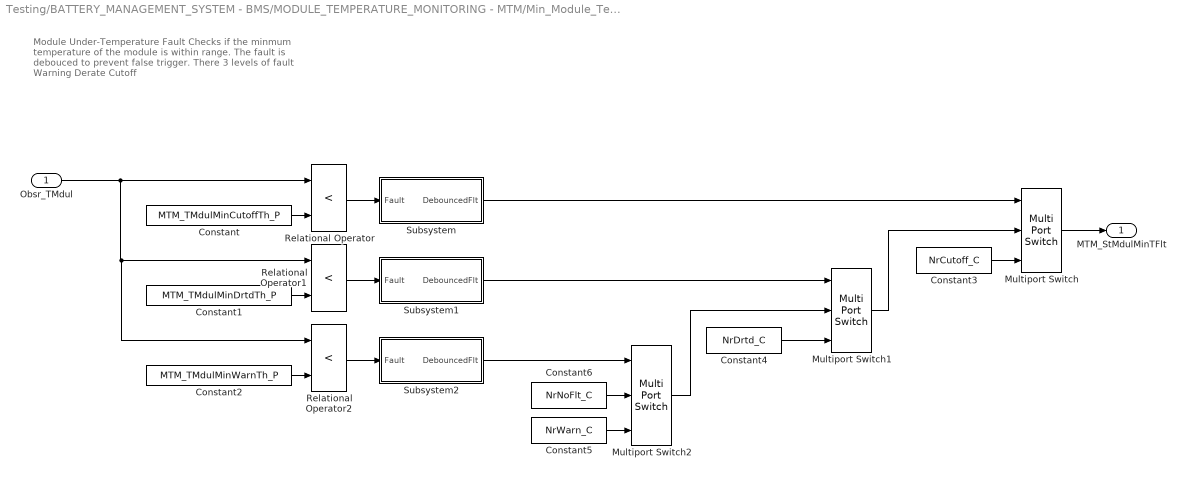
== system Testing/BATTERY_MANAGEMENT_SYSTEM - BMS/MODULE_TEMPERATURE_MONITORING - MTM/Min_Module_Temperature_Fault_State ==
  note: Module Under-Temperature Fault
      |
      | Checks if the minmum temperature of the module is within range. The fault is debouced to prevent false trigger.
      |
      | There 3 levels of fault
      | Warning
      | Derate
      | Cutoff
  Obsr_TMdul : Inport
  Constant : Constant  Value=MTM_TMdulMinCutoffTh_P
  Constant1 : Constant  Value=MTM_TMdulMinDrtdTh_P
  Constant2 : Constant  Value=MTM_TMdulMinWarnTh_P
  Constant3 : Constant  Value=NrCutoff_C
  Constant4 : Constant  Value=NrDrtd_C
  Constant5 : Constant  Value=NrWarn_C
  Constant6 : Constant  Value=NrNoFlt_C
  Multiport Switch : MultiPortSwitch  DataPortOrder=Zero-based contiguous  Inputs=2  zeroidx=on
  Multiport Switch1 : MultiPortSwitch  DataPortOrder=Zero-based contiguous  Inputs=2  zeroidx=on
  Multiport Switch2 : MultiPortSwitch  DataPortOrder=Zero-based contiguous  Inputs=2  zeroidx=on
  Relational Operator : RelationalOperator  Operator=<  OutDataTypeStr=boolean  RndMeth=Simplest
  Relational Operator1 : RelationalOperator  Operator=<  OutDataTypeStr=boolean  RndMeth=Simplest
  Relational Operator2 : RelationalOperator  Operator=<  OutDataTypeStr=boolean  RndMeth=Simplest
  Subsystem : Subsystem
  Subsystem1 : Subsystem
  Subsystem2 : Subsystem
  MTM_StMdulMinTFlt : Outport
  wires:
  Obsr_TMdul/1 -> Relational Operator2/1, Relational Operator1/1, Relational Operator/1
  Multiport Switch/1 -> MTM_StMdulMinTFlt/1
  Relational Operator/1 -> Subsystem/1(Fault)
  Constant/1 -> Relational Operator/2
  Multiport Switch1/1 -> Multiport Switch/2
  Constant3/1 -> Multiport Switch/3
  Relational Operator1/1 -> Subsystem1/1(Fault)
  Constant1/1 -> Relational Operator1/2
  Constant4/1 -> Multiport Switch1/3
  Multiport Switch2/1 -> Multiport Switch1/2
  Relational Operator2/1 -> Subsystem2/1(Fault)
  Constant2/1 -> Relational Operator2/2
  Constant5/1 -> Multiport Switch2/3
  Constant6/1 -> Multiport Switch2/2
  Subsystem/1(DebouncedFlt) -> Multiport Switch/1
  Subsystem1/1(DebouncedFlt) -> Multiport Switch1/1
  Subsystem2/1(DebouncedFlt) -> Multiport Switch2/1

== system Testing/BATTERY_MANAGEMENT_SYSTEM - BMS/CELL_VOLTAGE_MONITORING - CVM/Max_Cell_Voltage_Fault_State/Subsystem ==
  Fault : Inport
  Constant : Constant  Value=0
  Constant2 : Constant  Value=CVM_DMaxVCellMaxCutoff_P
  Constant3 : Constant  Value=CVM_DMinVCellMaxCutoff_P
  Subsystem : BMSLib/Debouncer
  DebouncedFlt : Outport
  wires:
  Fault/1 -> Subsystem/1
  Subsystem/1 -> DebouncedFlt/1
  [BMS_FltEnaFlag] -> Subsystem/2
  Constant/1 -> Subsystem/3
  Constant2/1 -> Subsystem/4
  Constant3/1 -> Subsystem/5

== system Testing/BATTERY_MANAGEMENT_SYSTEM - BMS/CELL_VOLTAGE_MONITORING - CVM/Max_Cell_Voltage_Fault_State/Subsystem1 ==
  Fault : Inport
  Constant1 : Constant  Value=0
  Constant2 : Constant  Value=CVM_DMaxVCellMaxDrtd_P
  Constant3 : Constant  Value=CVM_DMinVCellMaxDrtd_P
  Subsystem : BMSLib/Debouncer
  DebouncedFlt : Outport
  wires:
  Constant3/1 -> Subsystem/5
  Constant2/1 -> Subsystem/4
  Constant1/1 -> Subsystem/3
  [BMS_FltEnaFlag] -> Subsystem/2
  Subsystem/1 -> DebouncedFlt/1
  Fault/1 -> Subsystem/1

== system Testing/BATTERY_MANAGEMENT_SYSTEM - BMS/CELL_VOLTAGE_MONITORING - CVM/Max_Cell_Voltage_Fault_State/Subsystem2 ==
  Fault : Inport
  Constant1 : Constant  Value=0
  Constant2 : Constant  Value=CVM_DMaxVCellMaxWarn_P
  Constant3 : Constant  Value=CVM_DMinVCellMaxWarn_P
  Subsystem : BMSLib/Debouncer
  DebouncedFlt : Outport
  wires:
  Fault/1 -> Subsystem/1
  Subsystem/1 -> DebouncedFlt/1
  [BMS_FltEnaFlag] -> Subsystem/2
  Constant1/1 -> Subsystem/3
  Constant2/1 -> Subsystem/4
  Constant3/1 -> Subsystem/5

== system Testing/BATTERY_MANAGEMENT_SYSTEM - BMS/CELL_VOLTAGE_MONITORING - CVM/Min_Cell_Voltage_Fault_State/Subsystem ==
  Fault : Inport
  Constant1 : Constant  Value=0
  Constant2 : Constant  Value=CVM_DMaxVCellMinCutoff_P
  Constant3 : Constant  Value=CVM_DMinVCellMinCutoff_P
  Subsystem : BMSLib/Debouncer
  DebouncedFlt : Outport
  wires:
  Fault/1 -> Subsystem/1
  Subsystem/1 -> DebouncedFlt/1
  [BMS_FltEnaFlag] -> Subsystem/2
  Constant1/1 -> Subsystem/3
  Constant2/1 -> Subsystem/4
  Constant3/1 -> Subsystem/5

== system Testing/BATTERY_MANAGEMENT_SYSTEM - BMS/CELL_VOLTAGE_MONITORING - CVM/Min_Cell_Voltage_Fault_State/Subsystem1 ==
  Fault : Inport
  Constant1 : Constant  Value=0
  Constant2 : Constant  Value=CVM_DMaxVCellMinDrtd_P
  Constant3 : Constant  Value=CVM_DMinVCellMinDrtd_P
  Subsystem : BMSLib/Debouncer
  DebouncedFlt : Outport
  wires:
  Constant3/1 -> Subsystem/5
  Constant2/1 -> Subsystem/4
  Constant1/1 -> Subsystem/3
  [BMS_FltEnaFlag] -> Subsystem/2
  Subsystem/1 -> DebouncedFlt/1
  Fault/1 -> Subsystem/1

== system Testing/BATTERY_MANAGEMENT_SYSTEM - BMS/CELL_VOLTAGE_MONITORING - CVM/Min_Cell_Voltage_Fault_State/Subsystem2 ==
  Fault : Inport
  Constant1 : Constant  Value=0
  Constant2 : Constant  Value=CVM_DMaxVCellMinWarn_P
  Constant3 : Constant  Value=CVM_DMinVCellMinWarn_P
  Subsystem : BMSLib/Debouncer
  DebouncedFlt : Outport
  wires:
  Fault/1 -> Subsystem/1
  Subsystem/1 -> DebouncedFlt/1
  [BMS_FltEnaFlag] -> Subsystem/2
  Constant1/1 -> Subsystem/3
  Constant2/1 -> Subsystem/4
  Constant3/1 -> Subsystem/5

== system Testing/BATTERY_MANAGEMENT_SYSTEM - BMS/MODULE_TEMPERATURE_MONITORING - MTM/Max_Module_Temperature_Fault_State/Subsystem ==
  Fault : Inport
  Constant1 : Constant  Value=0
  Constant2 : Constant  Value=MTM_DMaxTMdulMaxCutoff_P
  Constant3 : Constant  Value=MTM_DMinTMdulMaxCutoff_P
  Subsystem : BMSLib/Debouncer
  DebouncedFlt : Outport
  wires:
  Fault/1 -> Subsystem/1
  Subsystem/1 -> DebouncedFlt/1
  [BMS_FltEnaFlag] -> Subsystem/2
  Constant1/1 -> Subsystem/3
  Constant2/1 -> Subsystem/4
  Constant3/1 -> Subsystem/5

== system Testing/BATTERY_MANAGEMENT_SYSTEM - BMS/MODULE_TEMPERATURE_MONITORING - MTM/Max_Module_Temperature_Fault_State/Subsystem1 ==
  Fault : Inport
  Constant1 : Constant  Value=0
  Constant2 : Constant  Value=MTM_DMaxTMdulMaxDrtd_P
  Constant3 : Constant  Value=MTM_DMinTMdulMaxDrtd_P
  Subsystem : BMSLib/Debouncer
  DebouncedFlt : Outport
  wires:
  Constant3/1 -> Subsystem/5
  Constant2/1 -> Subsystem/4
  Constant1/1 -> Subsystem/3
  [BMS_FltEnaFlag] -> Subsystem/2
  Subsystem/1 -> DebouncedFlt/1
  Fault/1 -> Subsystem/1

== system Testing/BATTERY_MANAGEMENT_SYSTEM - BMS/MODULE_TEMPERATURE_MONITORING - MTM/Max_Module_Temperature_Fault_State/Subsystem2 ==
  Fault : Inport
  Constant1 : Constant  Value=0
  Constant2 : Constant  Value=MTM_DMaxTMdulMaxWarn_P
  Constant3 : Constant  Value=MTM_DMinTMdulMaxWarn_P
  Subsystem : BMSLib/Debouncer
  DebouncedFlt : Outport
  wires:
  Fault/1 -> Subsystem/1
  Subsystem/1 -> DebouncedFlt/1
  [BMS_FltEnaFlag] -> Subsystem/2
  Constant1/1 -> Subsystem/3
  Constant2/1 -> Subsystem/4
  Constant3/1 -> Subsystem/5

== system Testing/BATTERY_MANAGEMENT_SYSTEM - BMS/MODULE_TEMPERATURE_MONITORING - MTM/Min_Module_Temperature_Fault_State/Subsystem ==
  Fault : Inport
  Constant1 : Constant  Value=0
  Constant2 : Constant  Value=MTM_DMaxTMdulMinCutoff_P
  Constant3 : Constant  Value=MTM_DMinTMdulMinCutoff_P
  Subsystem : BMSLib/Debouncer
  DebouncedFlt : Outport
  wires:
  Fault/1 -> Subsystem/1
  Subsystem/1 -> DebouncedFlt/1
  [BMS_FltEnaFlag] -> Subsystem/2
  Constant1/1 -> Subsystem/3
  Constant2/1 -> Subsystem/4
  Constant3/1 -> Subsystem/5

== system Testing/BATTERY_MANAGEMENT_SYSTEM - BMS/MODULE_TEMPERATURE_MONITORING - MTM/Min_Module_Temperature_Fault_State/Subsystem1 ==
  Fault : Inport
  Constant1 : Constant  Value=0
  Constant2 : Constant  Value=MTM_DMaxTMdulMinDrtd_P
  Constant3 : Constant  Value=MTM_DMinTMdulMinDrtd_P
  Subsystem : BMSLib/Debouncer
  DebouncedFlt : Outport
  wires:
  Constant3/1 -> Subsystem/5
  Constant2/1 -> Subsystem/4
  Constant1/1 -> Subsystem/3
  [BMS_FltEnaFlag] -> Subsystem/2
  Subsystem/1 -> DebouncedFlt/1
  Fault/1 -> Subsystem/1

== system Testing/BATTERY_MANAGEMENT_SYSTEM - BMS/MODULE_TEMPERATURE_MONITORING - MTM/Min_Module_Temperature_Fault_State/Subsystem2 ==
  Fault : Inport
  Constant1 : Constant  Value=0
  Constant2 : Constant  Value=MTM_DMaxTMdulMinWarn_P
  Constant3 : Constant  Value=MTM_DMinTMdulMinWarn_P
  Subsystem : BMSLib/Debouncer
  DebouncedFlt : Outport
  wires:
  Fault/1 -> Subsystem/1
  Subsystem/1 -> DebouncedFlt/1
  [BMS_FltEnaFlag] -> Subsystem/2
  Constant1/1 -> Subsystem/3
  Constant2/1 -> Subsystem/4
  Constant3/1 -> Subsystem/5

== matlab function Testing/MODE_STRING_FORMAT/MATLAB Function ==
  data: ModeNum input; BmsModeText output
function BmsModeText = BmsMode(ModeNum)
    if(ModeNum == 100)
        BmsModeText = [73 100 108 101 zeros(1,24)];
    elseif(ModeNum == 110)
        BmsModeText = [67 111 110 116 97 99 116 111 114 32 67 111 110 110 101 99 116 32 67 111 109 109 97 110 100 zeros(1,3)];
    elseif(ModeNum == 111)
        BmsModeText = [67 111 110 116 97 99 116 111 114 32 67 111 110 110 101 99 116 32 67 104 101 99 107 zeros(1,5)];
    elseif(ModeNum == 115)
        BmsModeText = [67 111 110 116 97 99 116 111 114 32 67 111 110 110 101 99 116 32 70 97 105 108 zeros(1,6)];
    elseif(ModeNum == 120)
        BmsModeText = [67 111 110 116 97 99 116 111 114 32 67 111 110 110 101 99 116 101 100 zeros(1,9)];
    elseif(ModeNum == 130)
        BmsModeText = [67 104 97 114 103 105 110 103 zeros(1,20)];
    elseif(ModeNum == 140)
        BmsModeText = [68 105 115 99 104 97 114 103 105 110 103 zeros(1,17)];
    elseif(ModeNum == 200)
        BmsModeText = [67 111 110 116 97 99 116 111 114 32 68 105 115 99 111 110 110 101 99 116 32 67 111 109 109 97 110 100];
    elseif(ModeNum == 211)
        BmsModeText = [67 111 110 116 97 99 116 111 114 32 68 105 115 99 111 110 110 101 99 116 32 67 104 101 99 107 zeros(1,2)];
    elseif(ModeNum == 230)
        BmsModeText = [67 111 110 116 97 99 116 111 114 32 68 105 115 99 111 110 110 101 99 116 32 70 97 105 108 zeros(1,3)];
    elseif(ModeNum == 240)
        BmsModeText = [67 111 110 116 97 99 116 111 114 32 68 105 115 99 111 110 110 101 99 116 32 83 117 99 99 101 115 115];
    else
        BmsModeText = [73 100 108 101 zeros(1,24)];
    end
end

== stateflow chart Testing/BATTERY_MANAGEMENT_SYSTEM - BMS/BATTERY_OPERATION_MODE - BM/BMS OPERATION MODE ==
  state IDLE
    entry:
    BM_OperMode = 100;
    BM_CtctrCnctCmd = false;
  state CONTACTOR_CONNECT_COMMAND
    entry:
    BM_OperMode = 110;
    BM_CtctrCnctCmd = true;
  state FAULT
    entry:
    BM_OperMode = 255;
    BM_CtctrCnctCmd = false;
  state CONTACTOR_CONNECT_FAIL
    entry:
    BM_OperMode = 115;
    BM_CtctrFlt = true;
  state CONTACTOR_CONNECT_CHECK
    entry:
    BM_OperMode = 111;
  state CONTACTOR_CONNECT_SEQUENCE1
    state CONTACTOR_CONNECT_SUCCESS
      entry:
      BM_OperMode = 120;
      BM_StsCtctrCnct = true;
    state CHARGING
      entry:
      BM_OperMode = 130;
    state DISCHARGING
      entry:
      BM_OperMode = 140;
    CONTACTOR_CONNECT_SEQUENCE1.CHARGING -> ? [order 2] : [(Obsr_StsChPlg == false)||(BPC_BattSoc >= 98.5 )]
    CONTACTOR_CONNECT_SEQUENCE1.DISCHARGING -> ? [order 2] : [((Obsr_StsIgnOn == false)||(BPC_BattSoc < 3 ))]
    CONTACTOR_CONNECT_SEQUENCE1.CONTACTOR_CONNECT_SUCCESS -> CONTACTOR_CONNECT_SEQUENCE1.CHARGING [order 1] : [Obsr_StsChPlg == true]
    CONTACTOR_CONNECT_SEQUENCE1.CONTACTOR_CONNECT_SUCCESS -> CONTACTOR_CONNECT_SEQUENCE1.DISCHARGING [order 2] : [Obsr_StsIgnOn == true]
    CONTACTOR_CONNECT_SEQUENCE1.DISCHARGING -> CONTACTOR_CONNECT_SEQUENCE1.CHARGING [order 1] : [Obsr_StsChPlg == true]
    CONTACTOR_CONNECT_SEQUENCE1.CHARGING -> CONTACTOR_CONNECT_SEQUENCE1.DISCHARGING [order 1] : [(Obsr_StsChPlg == false) && (Obsr_StsIgnOn == true)]
  state CONTACTOR_CONNECT_SEQUENCE
    state CONTACTOR_CONNECT_SUCCESS
      entry:
      BM_OperMode = 120;
      BM_StsCtctrCnct = true;
    state CHARGING
      entry:
      BM_OperMode = 130;
    state DISCHARGING
      entry:
      BM_OperMode = 140;
    CONTACTOR_CONNECT_SEQUENCE.CONTACTOR_CONNECT_SUCCESS -> CONTACTOR_CONNECT_SEQUENCE.CHARGING [order 1] : [Obsr_StsChPlg == true]
    CONTACTOR_CONNECT_SEQUENCE.CONTACTOR_CONNECT_SUCCESS -> CONTACTOR_CONNECT_SEQUENCE.DISCHARGING [order 2] : [Obsr_StsIgnOn == true]
    CONTACTOR_CONNECT_SEQUENCE.DISCHARGING -> CONTACTOR_CONNECT_SEQUENCE.CHARGING [order 1] : [Obsr_StsChPlg == true]
    CONTACTOR_CONNECT_SEQUENCE.CHARGING -> CONTACTOR_CONNECT_SEQUENCE.DISCHARGING [order 1] : [(Obsr_StsChPlg == false) && (Obsr_StsIgnOn == true)]
  state CONTACTOR_DICCONNECT_CHECK
    entry:
    BM_OperMode = 211;
  state CONTACTOR_DISCONNECT_FAIL
    entry:
    BM_OperMode = 230;
    BM_CtctrFlt = true;
  state CONTACTOR_DISCONNECT_COMMAND
    entry:
    BM_OperMode = 200;
    BM_CtctrCnctCmd = false;
  state CONTACTOR_DISCONNECT_SUCCESS
    entry:
    BM_OperMode = 220;
    BM_StsCtctrCnct = false;
  CONTACTOR_CONNECT_SEQUENCE.DISCHARGING -> CONTACTOR_DISCONNECT_COMMAND [order 2] : [((Obsr_StsIgnOn == false)||(BPC_BattSoc < 3 ))]
  CONTACTOR_CONNECT_SEQUENCE.CHARGING -> CONTACTOR_DISCONNECT_COMMAND [order 2] : [(Obsr_StsChPlg == false)||(BPC_BattSoc >= 98.5 )]
  (default) -> IDLE : {BM_CtctrFlt = false;
      | BM_StsCtctrCnct = false;}
  IDLE -> (junction 41) : [BFH_StsBattFlt == false]
  (junction 80) -> IDLE
  (junction 41) -> CONTACTOR_CONNECT_COMMAND : [((Obsr_StsIgnOn == true)&&(BPC_BattSoc > 3 ))||((Obsr_StsChPlg == true)&&(BPC_BattSoc < 98.5))]
  (junction 77) -> (junction 80)
  CONTACTOR_CONNECT_COMMAND -> CONTACTOR_CONNECT_CHECK : [after(BM_TiCtctrCnct_P,tick)]
  FAULT -> (junction 77) : [(Obsr_StsIgnOn == false) && (Obsr_StsChPlg == false)]
  (junction 96) -> (junction 77)
  CONTACTOR_CONNECT_FAIL -> FAULT
  CONTACTOR_CONNECT_CHECK -> CONTACTOR_CONNECT_FAIL [order 1] : [Obsr_VBus < 0.98*Obsr_VBatPack]
  CONTACTOR_DISCONNECT_FAIL -> FAULT
  CONTACTOR_DISCONNECT_SUCCESS -> FAULT [order 1] : [BFH_StsBattFlt == true]
  CONTACTOR_CONNECT_CHECK -> CONTACTOR_CONNECT_SEQUENCE.CONTACTOR_CONNECT_SUCCESS [order 2] : [Obsr_VBus >= 0.95*Obsr_VBatPack]
  CONTACTOR_CONNECT_SEQUENCE -> CONTACTOR_DISCONNECT_COMMAND : [BFH_StsBattFlt == true]
  CONTACTOR_DICCONNECT_CHECK -> CONTACTOR_DISCONNECT_FAIL [order 2]
  CONTACTOR_DISCONNECT_COMMAND -> CONTACTOR_DICCONNECT_CHECK : [after(BM_TiCtctrDCnct_P,tick)]
  CONTACTOR_DICCONNECT_CHECK -> CONTACTOR_DISCONNECT_SUCCESS [order 1] : [Obsr_VBus < 0.2*Obsr_VBatPack]
  CONTACTOR_DISCONNECT_SUCCESS -> (junction 96) [order 2]
  data: BFH_StsBattFlt input boolean; Obsr_StsIgnOn input boolean; Obsr_StsChPlg input boolean; BM_TiCtctrCnct_P input single; Obsr_VBus input single; Obsr_VBatPack input single; BM_TiCtctrDCnct_P input single; BM_OperMode output uint8; BM_CtctrFlt output boolean; BM_CtctrCnctCmd output boolean; BM_StsCtctrCnct output boolean; BPC_BattSoc input single
